simulink model "camera_radar_lidar"  (R2021b)
settings: Solver=FixedStepDiscrete  StartTime=0.0  StopTime=10.0  RelTol=1e-3
model workspace (MAT data in the model file):
  firstWarning = 1
  originalScenarioChecksum = 'D0B0A4B173DD3DA6100BB92ACC3E01B4'
undefined symbols (not defined in the file or in its folder): driving
libraries: drivingscenarioandsensors x7, sensorinslib x1
(part 1 of 22)
settings Model: Creator=ghisl  LastModifiedBy=ghisl

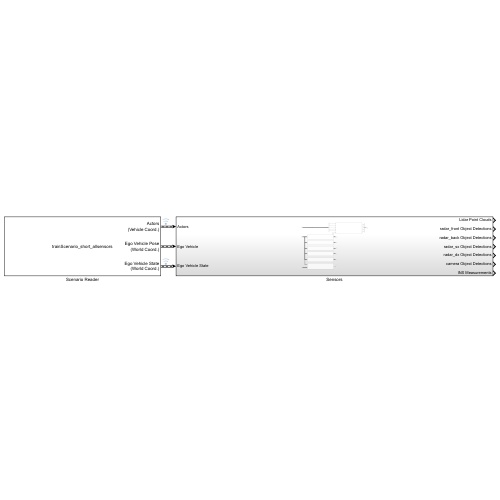
[thumbnail: Simulink's stored preview of the top-level diagram]
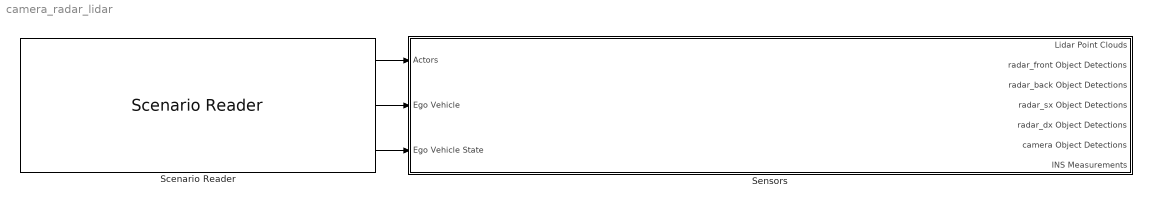
== system camera_radar_lidar ==
  Scenario Reader : drivingscenarioandsensors/Scenario Reader  ScenarioSource=From file  ScenarioFileName=G:\My Drive\UniBG\CORSI\Laurea Magistrale\2021_2022 - Magistrale Secondo Anno\secondo_semestre\Tirocinio Formativo\tirocinio_PRSE\matlab_stuff\object_recognition\obstacle_detection\camera_radar_lidar\trainScenario_short_allsensors.mat  ScenarioVariableName=scenario  OutputCoordinateSystem=Vehicle coordinates  EgoVehicleSource=Scenario  EgoVehicleActorID=1  OrientVehiclesOnRoad=off  OutputEgoVehiclePose=on  OutputEgoVehicleState=on  SampleTime=0.1  LaneBoundaryOutput=None  LaneBoundaryDistance=0:0.5:9.5  LaneBoundaryLocation=Center of lane markings  BusNameSource=Auto  BusName=BusActors  BusNumActorsSource=Scenario  BusNumActors=100  BusName2Source=Auto  BusName2=BusLaneBoundaries  BusNumLaneBoundariesSource=Scenario  BusNumLaneBoundaries=10  BusName3Source=Auto  BusName3=BusEgoActor  BusName4Source=Auto  BusName4=BusEgoState  ShowCoordinateLabels=on  SimulateUsing=Interpreted execution
  Sensors : Subsystem
  wires:
  Scenario Reader/1 -> Sensors/1(Actors)
  Scenario Reader/2 -> Sensors/2(Ego Vehicle)
  Scenario Reader/3 -> Sensors/3(Ego Vehicle State)
